simulink model "Vehicle_Following_Control"  (R2025b)
settings: Solver=VariableStepAuto  StartTime=0.0  StopTime=10.0  RelTol=1e-3
libraries: simulink x1
settings Model: Creator=Ceylin  LastModifiedBy=Ceylin

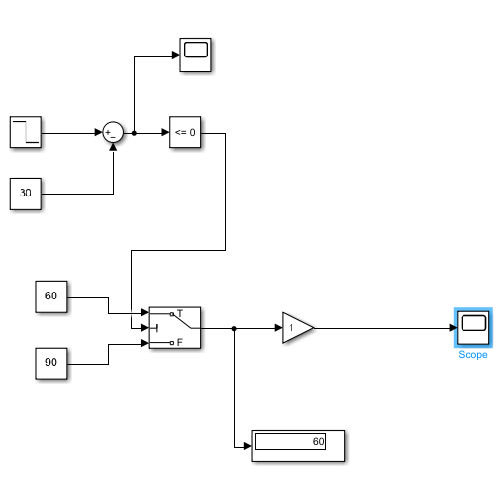
[thumbnail: Simulink's stored preview of the top-level diagram]
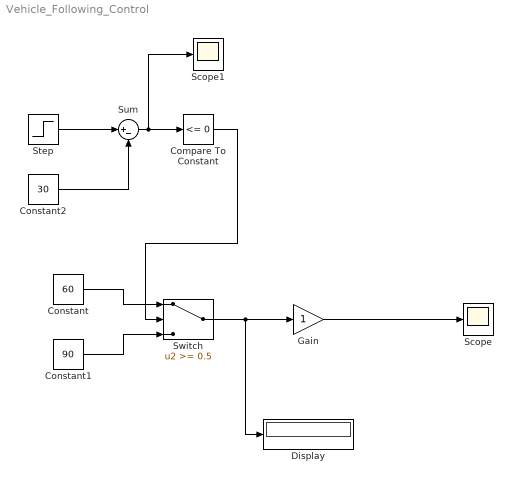
== system Vehicle_Following_Control ==
  Compare To Constant : simulink/Logic and Bit Operations/Compare To Constant  relop=<=  const=0  OutDataTypeStr=boolean
  Constant : Constant  Value=60
  Constant1 : Constant  Value=90
  Constant2 : Constant  Value=30
  Display : Display
  Gain : Gain
  Scope : Scope
      settings: ActiveDisplayYMinimum=56.25  ActiveDisplayYMaximum=93.75
  Scope1 : Scope
      settings: ActiveDisplayYMinimum=-12.5  ActiveDisplayYMaximum=12.5
  Step : Step  Time=5  Before=40  After=20  SampleTime=0
  Sum : Sum  Inputs=|+-
  Switch : Switch  Threshold=0.5  SaturateOnIntegerOverflow=off  InputSameDT=off
  wires:
  Constant/1 -> Switch/1
  Constant1/1 -> Switch/3
  Step/1 -> Sum/1
  Constant2/1 -> Sum/2
  Sum/1 -> Scope1/1, Compare To Constant/1
  Compare To Constant/1 -> Switch/2
  Switch/1 -> Display/1, Gain/1
  Gain/1 -> Scope/1
